simulink model "ej2a"  (R2021a)
settings: Solver=VariableStepAuto  StartTime=0.0  StopTime=10000  RelTol=1e-3
libraries: cstblocks x1
settings Model: Creator=franc  LastModifiedBy=franc

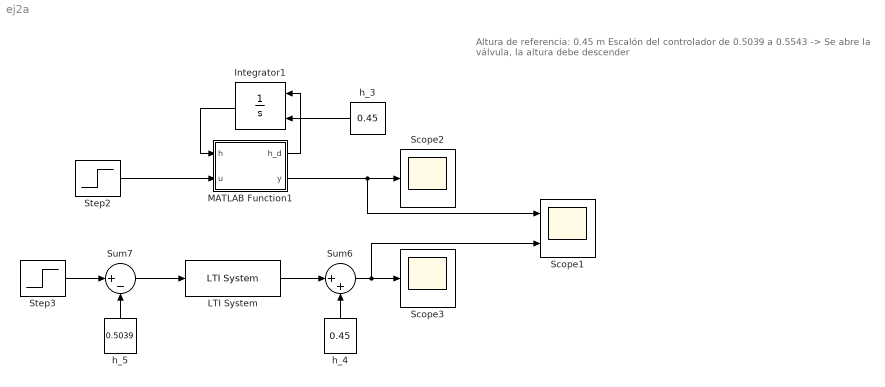
== system ej2a ==
  note: Altura de referencia: 0.45 m
      | Escalón del controlador de 0.5039 a 0.5543
      |
      | -> Se abre la válvula, la altura debe descender
  Integrator1 : Integrator  InitialConditionSource=external
  LTI System : cstblocks/LTI System  sys=planta  IC=[]
  MATLAB Function1 : MATLAB Function  TreatAsAtomicUnit=on
  Scope1 : Scope  NumInputPorts=2
  Scope2 : Scope
  Scope3 : Scope
  Step2 : Step  Before=0.5039  After=0.5543  SampleTime=0
  Step3 : Step  Before=0.5039  After=0.5543  SampleTime=0
  Sum6 : Sum  Inputs=|++
  Sum7 : Sum  Inputs=|+-
  h_3 : Constant  Value=0.45
  h_4 : Constant  Value=0.45
  h_5 : Constant  Value=0.5039
  wires:
  Sum6/1 -> Scope1/2, Scope3/1
  Step2/1 -> MATLAB Function1/2(u)
  h_3/1 -> Integrator1/2
  MATLAB Function1/2(y) -> Scope1/1, Scope2/1
  h_5/1 -> Sum7/2
  h_4/1 -> Sum6/2
  MATLAB Function1/1(h_d) -> Integrator1/1
  Integrator1/1 -> MATLAB Function1/1(h)
  Step3/1 -> Sum7/1
  Sum7/1 -> LTI System/1
  LTI System/1 -> Sum6/1

== matlab function ej2a/MATLAB Function1 ==
  data: h input; h_d output; u input; y output
function [h_d, y] = fcn(h, u)
    g = 9.8;        %En metros sobre segundo cuadrado
    H = 0.9;        %En metros
    L_s = 0.4;      %En metros
    L_i = 0.1;      %En metros
    Q_i = 0.0001333; %Metros cubicos por segundo
    d2 = 10.65e-3;
    A_o = pi * (d2 / 2)^2;

    h_d = (H^2 * (Q_i - A_o * sqrt(2*g*h)*u))/(h^2*(L_s-L_i)^2 + 2*h*L_i*(L_s-L_i)*H+L_i^2*H^2);
    y = h;
end
